simulink model "Hybrid_control_final"  (R2021a)
settings: Solver=ode4  StartTime=0.0  StopTime=2+dt  FixedStep=dt  RelTol=1e-3
settings Model: Creator=ravid  LastModifiedBy=Ashut
settings DebuggingCC: UnconnectedInputMsg=none  UnconnectedOutputMsg=none  UnconnectedLineMsg=none
settings RTWCC: DLArmComputeVersion=20.02.1

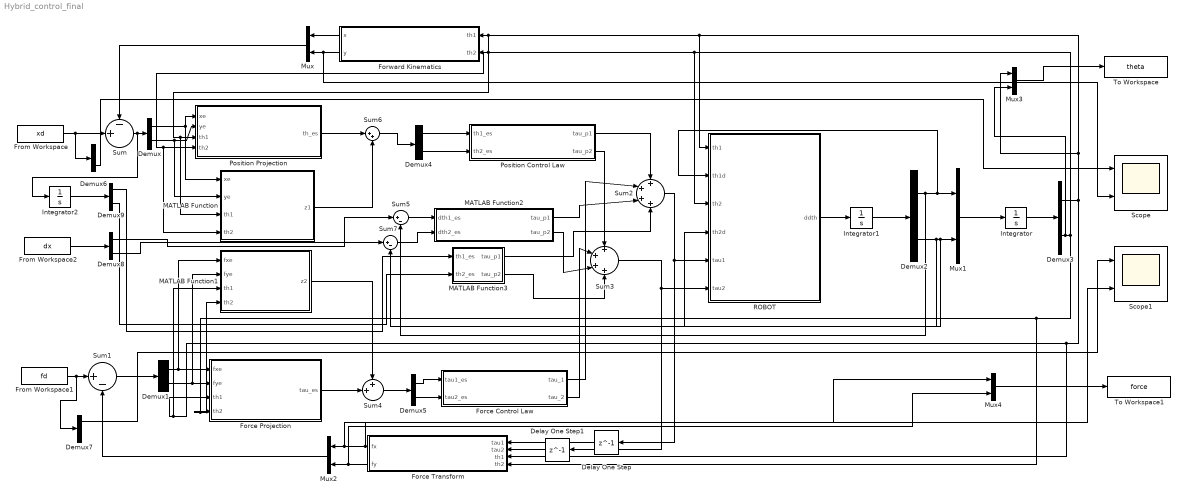
== system Hybrid_control_final ==
  Delay One Step : Delay  DelayLength=1
  Delay One Step1 : Delay  DelayLength=1
  Demux{,1..9} (10 alike) : Demux  Outputs=2
  Force Control Law : MATLAB Function  TreatAsAtomicUnit=on
  Force Projection : MATLAB Function  TreatAsAtomicUnit=on
  Force Transform : MATLAB Function  TreatAsAtomicUnit=on
  Forward Kinematics : MATLAB Function  TreatAsAtomicUnit=on
  From Workspace : FromWorkspace  VariableName=xd
  From Workspace1 : FromWorkspace  VariableName=fd
  From Workspace2 : FromWorkspace  VariableName=dx
  Integrator : Integrator  InitialCondition=[-pi/3;0]
  Integrator1 : Integrator  InitialCondition=[0;0]
  Integrator2 : Integrator
  MATLAB Function : MATLAB Function  TreatAsAtomicUnit=on
  MATLAB Function1 : MATLAB Function  TreatAsAtomicUnit=on
  MATLAB Function2 : MATLAB Function  TreatAsAtomicUnit=on
  MATLAB Function3 : MATLAB Function  TreatAsAtomicUnit=on
  Mux{,1..4} (5 alike) : Mux  Inputs=2
  Position Control Law : MATLAB Function  TreatAsAtomicUnit=on
  Position Projection : MATLAB Function  TreatAsAtomicUnit=on
  ROBOT : MATLAB Function  TreatAsAtomicUnit=on
  Scope : Scope  NumInputPorts=2
  Scope1 : Scope  NumInputPorts=2
  Sum : Sum  Inputs=-+|
  Sum1 : Sum  Inputs=|+-
  Sum2 : Sum  Inputs=++++
  Sum3 : Sum  Inputs=++++
  Sum4 : Sum  Inputs=++|
  Sum5 : Sum  Inputs=|+-
  Sum6 : Sum  Inputs=|++
  Sum7 : Sum  Inputs=|+-
  To Workspace : ToWorkspace  VariableName=theta  SaveFormat=Timeseries  SampleTime=-1
  To Workspace1 : ToWorkspace  VariableName=force  SaveFormat=Timeseries  SampleTime=-1
  wires:
  Position Control Law/1(tau_p1) -> Sum2/1
  Demux4/2 -> Position Control Law/2(th2_es)
  Demux4/1 -> Position Control Law/1(th1_es)
  Demux3/2 -> Mux3/2, Force Transform/4(th2), Force Projection/4(th2), MATLAB Function1/4(th2), MATLAB Function/4(th2), Position Projection/4(th2), Forward Kinematics/2(th2), ROBOT/3(th2)
  Mux1/1 -> Integrator/1
  Demux2/1 -> Sum5/2, ROBOT/2(th1d), Mux1/1
  Demux2/2 -> ROBOT/4(th2d), Mux1/2, Sum7/2
  Mux/1 -> Sum/1
  Demux3/1 -> Mux3/1, ROBOT/1(th1), MATLAB Function/3(th1), Position Projection/3(th1), Forward Kinematics/1(th1), Force Transform/3(th1), Force Projection/3(th1), MATLAB Function1/3(th1)
  Forward Kinematics/2(y) -> Scope/2, Mux/2
  Sum6/1 -> Demux4/1
  Demux/2 -> MATLAB Function/2(ye), Position Projection/2(ye)
  Demux/1 -> MATLAB Function/1(xe), Position Projection/1(xe)
  Sum/1 -> Integrator2/1, Demux/1
  Position Control Law/2(tau_p2) -> Sum3/1
  Forward Kinematics/1(x) -> Mux/1
  Integrator/1 -> Demux3/1
  ROBOT/1(ddth) -> Integrator1/1
  Force Control Law/2(tau_2) -> Sum3/2
  Position Projection/1(th_es) -> Sum6/1
  Force Control Law/1(tau_1) -> Sum2/2
  Integrator1/1 -> Demux2/1
  From Workspace1/1 -> Demux7/1, Sum1/1
  From Workspace/1 -> Demux6/1, Sum/2
  MATLAB Function/1(z1) -> Sum6/2
  Sum2/1 -> Delay One Step/1, ROBOT/5(tau1)
  Sum3/1 -> Delay One Step1/1, ROBOT/6(tau2)
  Demux1/1 -> MATLAB Function1/1(fxe), Force Projection/1(fxe)
  Demux1/2 -> MATLAB Function1/2(fye), Force Projection/2(fye)
  Sum1/1 -> Demux1/1
  MATLAB Function1/1(z2) -> Sum4/1
  Force Projection/1(tau_es) -> Sum4/2
  Demux5/1 -> Force Control Law/1(tau1_es)
  Demux5/2 -> Force Control Law/2(tau2_es)
  Sum4/1 -> Demux5/1
  Force Transform/1(fx) -> Scope1/2, Mux4/1, Mux2/1
  Force Transform/2(fy) -> Mux4/2, Mux2/2
  Mux2/1 -> Sum1/2
  Delay One Step/1 -> Force Transform/1(tau1)
  Delay One Step1/1 -> Force Transform/2(tau2)
  Demux6/2 -> Scope/1
  Demux7/1 -> Scope1/1
  Mux3/1 -> To Workspace/1
  Mux4/1 -> To Workspace1/1
  MATLAB Function2/1(tau_p1) -> Sum2/3
  MATLAB Function2/2(tau_p2) -> Sum3/3
  From Workspace2/1 -> Demux8/1
  Sum5/1 -> MATLAB Function2/1(dth1_es)
  Sum7/1 -> MATLAB Function2/2(dth2_es)
  Demux8/1 -> Sum5/1
  Demux8/2 -> Sum7/1
  MATLAB Function3/1(tau_p1) -> Sum2/4
  MATLAB Function3/2(tau_p2) -> Sum3/4
  Demux9/1 -> MATLAB Function3/1(th1_es)
  Demux9/2 -> MATLAB Function3/2(th2_es)
  Integrator2/1 -> Demux9/1

== matlab function Hybrid_control_final/MATLAB Function2 ==
  data: dth1_es input; tau_p1 output; dth2_es input; tau_p2 output
function [tau_p1,tau_p2] = velocity_control_law(dth1_es,dth2_es)

%Kp1= 50;
% Ki1 = 0.01;
Kd = 1;
% s = tf('s');


tau_p1 =  Kd*(dth1_es); %+ Ki1*(th1_es)/s + Kd*(th1_es)*s;
tau_p2 =  Kd*(dth2_es); %+ Ki1*(th2_es)/s + Kd*(th2_es)*s;

== matlab function Hybrid_control_final/MATLAB Function3 ==
  data: th1_es input; tau_p1 output; th2_es input; tau_p2 output
function [tau_p1,tau_p2] = Integral_control_law(th1_es,th2_es)

KI= 0.01;
% Ki1 = 0.01;
%kd = 0.1;
% s = tf('s');


tau_p1 =  KI*(th1_es); %+ Ki1*(th1_es)/s + Kd*(th1_es)*s;
tau_p2 =  KI*(th2_es); %+ Ki1*(th2_es)/s + Kd*(th2_es)*s;

== matlab function Hybrid_control_final/Force Projection ==
  data: fxe input; tau_es output; fye input; th1 input; th2 input
function tau_es = Force_Projection(fxe,fye,th1,th2)


S = [1 0;0 0];

l1=1;l2=1;

J=[-l1*sin(th1) - l2*sin(th1+th2),-l2*sin(th1+th2);l1*cos(th1)+l2*cos(th1+th2),l2*cos(th1+th2)];

f_es = [fxe;fye];

tau_es = (S*J)'*f_es;

== matlab function Hybrid_control_final/Position Projection ==
  data: xe input; th_es output; ye input; th1 input; th2 input
function th_es = Position_Projection(xe,ye,th1,th2)

S = [0 0;0 1];

l1=1;l2=1;

J=[-l1*sin(th1) - l2*sin(th1+th2),-l2*sin(th1+th2);l1*cos(th1)+l2*cos(th1+th2),l2*cos(th1+th2)];

x_es = [xe;ye];

th_es = pinv(S*J)*x_es;

== matlab function Hybrid_control_final/Position Control Law ==
  data: th1_es input; tau_p1 output; tau_p2 output; th2_es input
function [tau_p1,tau_p2] = position_control_law(th1_es,th2_es)

Kp1= 5;
% Ki1 = 0.01;
%kd = 0.1;
% s = tf('s');


tau_p1 =  Kp1*(th1_es); %+ Ki1*(th1_es)/s + Kd*(th1_es)*s;
tau_p2 =  Kp1*(th2_es); %+ Ki1*(th2_es)/s + Kd*(th2_es)*s;

== matlab function Hybrid_control_final/Force Control Law ==
  data: tau1_es input; tau_1 output; tau_2 output; tau2_es input
function [tau_1,tau_2] = force_control_law(tau1_es,tau2_es)


Kp1= 1;
% Ki1 = 0.01;
% Kd = 0.1;

tau_1 =  Kp1*(tau1_es); %+ Ki1*(tau1_es)/s + Kd*(tau1_es)*s;
tau_2 =  Kp1*(tau2_es); %+ Ki1*(tau2_es)/s + Kd*(tau2_es)*s;

== matlab function Hybrid_control_final/ROBOT ==
  data: th1 input; ddth output; th1d input; th2 input; th2d input; tau1 input; tau2 input
function ddth= ode_solver_script_q1_a(th1,th1d,th2,th2d,tau1,tau2)
x = [th1;th1d;th2;th2d];
%% Input parameters
m2=1; m1=1; l1=1; l2=1; g=9.81;


%% Equation of motion 

%M matrix
M11=((((m1/3) + m2)*l1^2) +((m2/3)*l2^2) + (m2*l1*l2*cos(x(3))));
M12=(m2*(((l2^2)/3) + (0.5*l1*l2*cos(x(3)))));
M21=M12;
M22=((1/3)*m2*l2*l2);

%H matrix
H1 =((-m2*l1*l2*sin(x(3))*x(2)*x(4)) - (0.5*m2*l1*l2*sin(x(3))*x(4)*x(4)));
H2 = (0.5 * m2* l1*l2*sin(x(3))*x(2)*x(2));

%G matrix
G1=( ((((0.5*m1) + m2)*l1*cos(x(1))) + (0.5*m2*l2*cos(x(1)+x(3))))*g);
G2=0.5*m2*l2*cos(x(1)+x(3))*g;



M=[M11 M12;M21 M22];

HG = [H1 + G1; H2 + G2];

T=[tau1; tau2];

%% Equation in terms of acceleration

ddth = (inv(M)) * (T)    ;% Joint  accelaration

== matlab function Hybrid_control_final/Forward Kinematics ==
  data: x output; th1 input; y output; th2 input
function [x,y] = Foward_Kinematics(th1,th2)

l1=1;l2=1;
x=l1*cos(th1) + l2*cos(th1+ th2);
y=l1*sin(th1) + l2*sin(th1+ th2);

== matlab function Hybrid_control_final/Force Transform ==
  data: tau1 input; fx output; tau2 input; fy output; th1 input; th2 input
function [fx,fy] = Force_Transform(tau1,tau2,th1,th2)

l1=1;l2=1;

J=[-l1*sin(th1) - l2*sin(th1+th2),-l2*sin(th1+th2);l1*cos(th1)+l2*cos(th1+th2),l2*cos(th1+th2)];

tau = [tau1;tau2];

f = pinv(J')*tau;

fx = f(1);
fy = f(2);

== matlab function Hybrid_control_final/MATLAB Function ==
  data: xe input; ye input; z1 output; th1 input; th2 input
function z1 = null_projection(xe,ye,th1,th2)

xes = [xe;ye];
l1=1;l2=1;

J=[-l1*sin(th1) - l2*sin(th1+th2),-l2*sin(th1+th2);l1*cos(th1)+l2*cos(th1+th2),l2*cos(th1+th2)];

I = [1 0; 0 1];

z_th = pinv(J)*xes;

z1 = (I - (pinv(J)*J))*z_th;

== matlab function Hybrid_control_final/MATLAB Function1 ==
  data: fxe input; z2 output; fye input; th1 input; th2 input
function z2 = null_projection(fxe,fye,th1,th2)

fes = [fxe;fye];
l1=1;l2=1;

J=[-l1*sin(th1) - l2*sin(th1+th2),-l2*sin(th1+th2);l1*cos(th1)+l2*cos(th1+th2),l2*cos(th1+th2)];

I = [1 0; 0 1];

z_tau = pinv(J)*fes;

z2 = (I - (pinv(J)*J))*z_tau;
